simulink model "AFASClosedloopSim"  (R2023a)
settings: Solver=FixedStepAuto  StartTime=0.0  StopTime=600  FixedStep=1/240  RelTol=1e-5
PreLoadFcn:
  | [aircraft, state] = astDehavillandBeaver();
  | thrustX = getCoefficient(aircraft,"CX","Propeller",Component="Propeller");
InitFcn:
  | AFASClosedloopSimInitialization
model workspace (MATLAB code in the model file + MAT data in the model file):
  AirReferencedVelocity = 1
  AircraftPerformance : object (value not decoded)
  CurrentWaypoint = 1
  FCCLatDirMode = 1
  FCCVerticalMode = 1
  FlightPlan = 1
  LookaheadDis = 15
  NextWaypoint = 1
  NumofWaypoint = 1
  OwnshipAircraftID = 1
  PreWaypoint = 1
  PreviousWaypoint : Simulink.Parameter (value not decoded)
  TrajectoryChange = 1
  WaypointType = 1
  inputs0 : object (value not decoded)
  states : object (value not decoded)
  states0 : object (value not decoded)
  other statements: initialize6DOFSkyHogg;
values from neighbouring files (symbols this model uses):
  alt_ft = 1000    [AFASClosedloopSimInitialization.m]
  alt_hold_av = 1.5    [AFASClosedloopSimInitialization.m]
  alt_hold_hold = 0.1    [AFASClosedloopSimInitialization.m]
  alt_hold_vs = 0.58    [AFASClosedloopSimInitialization.m]
  alt_m = 304.8    [AFASClosedloopSimInitialization.m]
  AT_lead_T1 = 1    [AFASClosedloopSimInitialization.m]
  AT_lead_T2 = 1    [AFASClosedloopSimInitialization.m]
  AT_spd_hold_cmpst = 0.5    [AFASClosedloopSimInitialization.m]
  AT_spd_hold_ptch_tau_gain = 0.15    [AFASClosedloopSimInitialization.m]
  AT_spd_hold_rate_damping_gain = 10    [AFASClosedloopSimInitialization.m]
  AT_spd_hold_tas_lp_tau = 5.0    (= 5)    [AFASClosedloopSimInitialization.m]
  AT_spd_hold_tas_val_lp_tau = 0.5    [AFASClosedloopSimInitialization.m]
  AT_struct_den = 1    [AFASClosedloopSimInitialization.m]
  AT_struct_num = 1    [AFASClosedloopSimInitialization.m]
  AT_svo_composite = 1    [AFASClosedloopSimInitialization.m]
  av_hp_fltr_tau = 10    [AFASClosedloopSimInitialization.m]
  av_lp_fltr_tau = 0.5    [AFASClosedloopSimInitialization.m]
  cas_mps = 72.0222    [AFASClosedloopSimInitialization.m]
  Cl0 = 5.910000000000000e-04    (= 0.000591)    [AFASClosedloopSimInitialization.m]
  Cl_beta = -0.0618    [AFASClosedloopSimInitialization.m]
  Cl_da = -0.0992    [AFASClosedloopSimInitialization.m]
  Cl_da_alpha = -0.0827    [AFASClosedloopSimInitialization.m]
  Cl_dr = 0.0069    [AFASClosedloopSimInitialization.m]
  Cl_p = -0.5045    [AFASClosedloopSimInitialization.m]
  Cl_r = 0.1695    [AFASClosedloopSimInitialization.m]
  Cm0 = 0.0945    [AFASClosedloopSimInitialization.m]
  Cm_alpha = -0.6028    [AFASClosedloopSimInitialization.m]
  Cm_alpha2 = -2.1400    (= -2.14)    [AFASClosedloopSimInitialization.m]
  Cm_beta2 = 0.6921    [AFASClosedloopSimInitialization.m]
  Cm_de = -1.9210    (= -1.921)    [AFASClosedloopSimInitialization.m]
  Cm_df = 0.4072    [AFASClosedloopSimInitialization.m]
  Cm_q = -15.5600    (= -15.56)    [AFASClosedloopSimInitialization.m]
  Cm_r = -0.3118    [AFASClosedloopSimInitialization.m]
  Cn0 = -0.0031    [AFASClosedloopSimInitialization.m]
  Cn_beta = 0.0067    [AFASClosedloopSimInitialization.m]
  Cn_beta3 = 0.1373    [AFASClosedloopSimInitialization.m]
  Cn_da = -0.0039    [AFASClosedloopSimInitialization.m]
  Cn_dr = -0.0827    [AFASClosedloopSimInitialization.m]
  Cn_p = -0.1585    [AFASClosedloopSimInitialization.m]
  Cn_q = 0.1595    [AFASClosedloopSimInitialization.m]
  Cn_r = -0.1112    [AFASClosedloopSimInitialization.m]
  Cx0 = -0.0355    [AFASClosedloopSimInitialization.m]
  Cx_alpha = 0.0029    [AFASClosedloopSimInitialization.m]
  Cx_alpha2 = 5.4590    (= 5.459)    [AFASClosedloopSimInitialization.m]
  Cx_alpha3 = -5.1620    (= -5.162)    [AFASClosedloopSimInitialization.m]
  Cx_df = -0.0945    [AFASClosedloopSimInitialization.m]
  Cx_df_alpha = 1.1060    (= 1.106)    [AFASClosedloopSimInitialization.m]
  Cx_dr = 0.0341    [AFASClosedloopSimInitialization.m]
  Cx_q = -0.6748    [AFASClosedloopSimInitialization.m]
  Cy0 = -0.0022    [AFASClosedloopSimInitialization.m]
  Cy_beta = -0.7678    [AFASClosedloopSimInitialization.m]
  Cy_da = -0.0296    [AFASClosedloopSimInitialization.m]
  Cy_dr = 0.1158    [AFASClosedloopSimInitialization.m]
  Cy_dr_alpha = 0.5238    [AFASClosedloopSimInitialization.m]
  Cy_p = -0.1240    (= -0.124)    [AFASClosedloopSimInitialization.m]
  Cy_r = 0.3666    [AFASClosedloopSimInitialization.m]
  Cz0 = -0.0550    (= -0.055)    [AFASClosedloopSimInitialization.m]
  Cz_alpha = -5.5780    (= -5.578)    [AFASClosedloopSimInitialization.m]
  Cz_alpha3 = 3.4420    (= 3.442)    [AFASClosedloopSimInitialization.m]
  Cz_de = -0.3980    (= -0.398)    [AFASClosedloopSimInitialization.m]
  Cz_de_beta = -15.9300    (= -15.93)    [AFASClosedloopSimInitialization.m]
  Cz_df = -1.3770    (= -1.377)    [AFASClosedloopSimInitialization.m]
  Cz_df_alpha = -1.2610    (= -1.261)    [AFASClosedloopSimInitialization.m]
  Cz_q = -2.9880    (= -2.988)    [AFASClosedloopSimInitialization.m]
  hdg_select_hdg_rate_capt = 0.2    [AFASClosedloopSimInitialization.m]
  hdg_select_hdg_rate_damping = 1    [AFASClosedloopSimInitialization.m]
  hdg_select_hdg_rate_track = 0.05    [AFASClosedloopSimInitialization.m]
  lat_accel_aug_lp_tau = 10    [AFASClosedloopSimInitialization.m]
  ltrl_acc_gain = -0.04    [AFASClosedloopSimInitialization.m]
  ltrl_acc_lp_tau = 0.5    [AFASClosedloopSimInitialization.m]
  mach = 0.213    [AFASClosedloopSimInitialization.m]
  OwnshipAircraftConfig = 0    [AFASClosedloopSimInitialization.m]
  pitch_att_gain = 0.7    [AFASClosedloopSimInitialization.m]
  pitch_lead_T1 = 1    [AFASClosedloopSimInitialization.m]
  pitch_lead_T2 = 1    [AFASClosedloopSimInitialization.m]
  pitch_rate_gain = -1400    [AFASClosedloopSimInitialization.m]
  pitch_rate_gain_GAIN1 = -56    [AFASClosedloopSimInitialization.m]
  pitch_rate_gain_GAIN2 = -52.25    [AFASClosedloopSimInitialization.m]
  pitch_rate_gain_IAS1 = 100    [AFASClosedloopSimInitialization.m]
  pitch_rate_gain_IAS2 = 380    [AFASClosedloopSimInitialization.m]
  pitch_rate_gain_schd = [4.24        2.80        2.24        1.68        1.44        1.22        0.97        0.85        0.77        0.72        0.66    ] * 1000    [AFASClosedloopSimInitialization.m]
  pitch_rate_gain_spd = [85          100.0       120.00      140.00      160.00      180.00      200.00      220.00      240.00      260.00      275.00  ] * 0.5144444    [AFASClosedloopSimInitialization.m]
  pitch_schedule_type = 3    [AFASClosedloopSimInitialization.m]
  pitch_struct_den = 1    [AFASClosedloopSimInitialization.m]
  pitch_struct_num = 1    [AFASClosedloopSimInitialization.m]
  pitch_svo_composite = 1    [AFASClosedloopSimInitialization.m]
  pitch_svo_integral = 0.6    [AFASClosedloopSimInitialization.m]
  roll_att_gain = 0.45    [AFASClosedloopSimInitialization.m]
  roll_lead_T1 = 1    [AFASClosedloopSimInitialization.m]
  roll_lead_T2 = 1    [AFASClosedloopSimInitialization.m]
  roll_limit = 30*d2r    (= 0.5235987)    [AFASClosedloopSimInitialization.m]
  roll_rate_gain = 561.5    [AFASClosedloopSimInitialization.m]
  roll_rate_gain_GAIN1 = 57.25    [AFASClosedloopSimInitialization.m]
  roll_rate_gain_GAIN2 = 41.25    [AFASClosedloopSimInitialization.m]
  roll_rate_gain_IAS1 = 100    [AFASClosedloopSimInitialization.m]
  roll_rate_gain_IAS2 = 380    [AFASClosedloopSimInitialization.m]
  roll_rate_gain_schd = [1.30        0.86        0.71        0.63        0.57        0.50        0.46        0.46    ] * 1000    [AFASClosedloopSimInitialization.m]
  roll_rate_gain_spd = [85.00       100.00      120.00      140.00      160.00      200.00      220.00      275.00  ] * 0.5144444    [AFASClosedloopSimInitialization.m]
  roll_schedule_type = 3    [AFASClosedloopSimInitialization.m]
  roll_struct_den = 1    [AFASClosedloopSimInitialization.m]
  roll_struct_num = 1    [AFASClosedloopSimInitialization.m]
  roll_svo_composite = 0.00001    (= 1e-05)    [AFASClosedloopSimInitialization.m]
  roll_svo_integral = 0.6    [AFASClosedloopSimInitialization.m]
  tas_mps = 73.051    [AFASClosedloopSimInitialization.m]
  TGR = 0.25    [AFASClosedloopSimInitialization.m]
  wingrock_enable_alt = 20000    [AFASClosedloopSimInitialization.m]
  wingrock_enable_mach = 0.6    [AFASClosedloopSimInitialization.m]
  wingrock_lookup_data = [2 2  1 1]    [AFASClosedloopSimInitialization.m]
  wingrock_lookup_row = [0 2 5 10]*pi/180    [AFASClosedloopSimInitialization.m]
  wingrock_schedule_type = 3    [AFASClosedloopSimInitialization.m]
  yaw_rate_gain = 15521    [AFASClosedloopSimInitialization.m]
  yaw_rate_gain_GAIN1 = 37.8352    [AFASClosedloopSimInitialization.m]
  yaw_rate_gain_GAIN2 = 24.2654    [AFASClosedloopSimInitialization.m]
  yaw_rate_gain_IAS1 = 100    [AFASClosedloopSimInitialization.m]
  yaw_rate_gain_IAS2 = 340    [AFASClosedloopSimInitialization.m]
  yaw_rate_gain_piecewise_schd = [7.68	5.98		3.22	2.59		1.78 ... (first row only)    [AFASClosedloopSimInitialization.m]
  yaw_rate_gain_schd = [15521    11532   11532   10115   8951.7  7831.7  6829.2  5739.3  4506.7  3317.9  3391.5  2103.9  1404.5  994.3226]    [AFASClosedloopSimInitialization.m]
  yaw_rate_gain_spd = [90       97      106     111     118     127     136     149     165     187     192     228     264     295     ] * 0.5144444    [AFASClosedloopSimInitialization.m]
  yaw_rate_hp_tau = 1.8    [AFASClosedloopSimInitialization.m]
  yd_lead_T1 = yd_a * yd_lead_T2    [AFASClosedloopSimInitialization.m]
  ... (+7 more)
undefined symbols (not defined in the file or in its folder): aircraft, DiscIntNeverNeededParam, Earth, F, Light, MIL, sigbuilder_block, state, WGS84
libraries: aerolibasang x4, aerolibactuator x4, aerolibguid x2, simulink x2, dspnetwork x2, etargetslib x2, shared6dof x1, aerolibadyn x1, aerolibatmos2 x1, aerolibwind2 x1, aerolibtransform2 x1, sharedtransform x1
(part 2 of 4)

== system AFASClosedloopSim/FMGC (Flight Mgt and Guidance & Control)/AFCC: Albatross.ai Flight Control Computer ==
  TMTargets : Inport
  RMTargets : Inport  Port=2
  OwnshipStates : Inport  Port=3
  Bus Selector : BusSelector  OutputSignals=SpdTarget,AltTarget
  Constant : Constant  Value=FCCVerticalMode
  Constant1 : Constant  Value=FCCLatDirMode
  FCC: Mode Logic and Behavior Logic : Subsystem
  FCC: Outerloop & Innerloop Control Laws : Subsystem
  ATServoCmd : Outport
  PitchServoCmd : Outport  Port=2
  RollServoCmd : Outport  Port=3
  YawServoCmd : Outport  Port=4
  wires:
  FCC: Outerloop & Innerloop Control Laws/1(ATServoCmd) -> ATServoCmd/1
  FCC: Outerloop & Innerloop Control Laws/2(PitchServoCmd) -> PitchServoCmd/1
  FCC: Outerloop & Innerloop Control Laws/3(RollSevoCmd) -> RollServoCmd/1
  TMTargets/1 -> Bus Selector/1
  RMTargets/1 -> FCC: Mode Logic and Behavior Logic/3(HDGTarget)
  Bus Selector/1 -> FCC: Mode Logic and Behavior Logic/1(SpdTarget)  "<SpdTarget>"
  Bus Selector/2 -> FCC: Mode Logic and Behavior Logic/2(AltTarget)  "<AltTarget>"
  Constant/1 -> FCC: Mode Logic and Behavior Logic/4(FCCVerticalMode)
  Constant1/1 -> FCC: Mode Logic and Behavior Logic/5(FCCLatDirMode)
  FCC: Mode Logic and Behavior Logic/1(SpdTargetLimited) -> FCC: Outerloop & Innerloop Control Laws/1(SpdTargetLimited)
  FCC: Mode Logic and Behavior Logic/2(AltTargetLimited) -> FCC: Outerloop & Innerloop Control Laws/2(AltTargetLimited)
  FCC: Mode Logic and Behavior Logic/3(HDGTargetLimited) -> FCC: Outerloop & Innerloop Control Laws/3(HDGTargetLimited)
  FCC: Outerloop & Innerloop Control Laws/4(YawServoCmd) -> YawServoCmd/1
  OwnshipStates/1 -> FCC: Outerloop & Innerloop Control Laws/4(OwnshipStates)

== system AFASClosedloopSim/FMGC (Flight Mgt and Guidance & Control)/AFMS: Albatross Flight Management System ==
  OwnshipStates : Inport
  4DTCmd : Inport  Port=2
  Add : Sum  Inputs=+-
  Add1 : Sum  Inputs=+-
  Add2 : Sum  Inputs=+-
  Bus Creator : BusCreator  Inputs=2
  Bus Selector : BusSelector  OutputSignals=Xe,Ye,Ze,u,v,w,psi
  C Caller : CCaller  FunctionName=add  PortSpecificationStruct="%)30     .    6 4   8    (     @         %    \"     ,    !     0         %  0 \"0    $    _    07)G3F%M90  4&]R=$YA;64 4V-O<&4     26YD97@     5'EP90      4VEZ90      27-';&]B86P   X    P    !@    @    $          4    (     0    ,    !         !   P!O=70 #@   #     &    \"     0         !0    @    !     P    $         $  # &]U=  .    .     8    (    !          %    \"     $    &     0         0    !@   $]U='!U=   #@   #@    &    \"     8         !0    @    !     0    $         \"0    @               X    X    !@    @    $          4    (     0    8    !         !     &    9&]U8FQE   .    ,     8    (    !          %    \"     $    !     0         0  $ ,0    X    P    !@    @    ) @        4    (     0    $    !          (  0      #@   #     &    \"     0         !0    @    !     @    $         $  \" '4Q   .    ,     8    (    !          %    \"     $    \"     0         0  ( =3$   X    X    !@    @    $          4    (     0    4    !         !     %    26YP=70    .    .     8    (    !@         %    \"     $    !     0         )    \"               #@   #@    &    \"     0         !0    @    !    !@    $         $     8   !D;W5B;&4   X    P    !@    @    $          4    (     0    $    !         !   0 Q    #@   #     &    \"     D\"        !0    @    !     0    $          @ !       .    ,     8    (    !          %    \"     $    \"     0         0  ( =3(   X    P    !@    @    $          4    (     0    (    !         !   @!U,@  #@   #@    &    \"     0         !0    @    !    !0    $         $     4   !);G!U=     X    X    !@    @    &          4    (     0    $    !          D    (            \\#\\.    .     8    (    !          %    \"     $    &     0         0    !@   &1O=6)L90  #@   #     &    \"     0         !0    @    !     0    $         $  ! #$    .    ,     8    (    \"0(        %    \"     $    !     0         \"  $"
  Calculate Range : aerolibguid/Calculate Range
  Constant : Constant
  Constant1 : Constant
  Current Time : DigitalClock
  CurrentWP : Constant  Value=[117.28257863691368,39.22176648931558,527.0,600]
  Demux : Demux
  Divide : Product  Inputs=*/
  Gain : Gain  Gain=-1
  Mux1 : Mux  Inputs=3
  Mux2 : Mux  Inputs=3
  Scope : Scope
  Scope1 : Scope
  Scope2 : Scope  NumInputPorts=7
  Selector1 : Selector  IndexMode=Zero-based  InputPortWidth=16  IndexOptions=Index vector (port)  Indices=[1]  OutputSizes=1
  Terminator : Terminator
  Trigonometric Function : Trigonometry  Operator=atan2
  WGS84_Location : Subsystem
  TMTargets : Outport
  RMTargets : Outport  Port=2
  wires:
  WGS84_Location/1(x) -> Mux1/1, Add2/1
  OwnshipStates/1 -> Bus Selector/1
  Demux/1 -> WGS84_Location/1(lon)  "<LONGWGS84>"
  Constant/1 -> C Caller/1
  CurrentWP/1 -> Demux/1
  C Caller/1 -> Selector1/2
  Constant1/1 -> C Caller/2
  Demux/2 -> WGS84_Location/2(lat)
  Demux/3 -> Gain/1
  Demux/4 -> Add/1
  Current Time/1 -> Add/2
  Add1/1 -> Trigonometric Function/1
  WGS84_Location/2(y) -> Add1/1, Mux1/2
  Gain/1 -> Bus Creator/2, Mux1/3  "AltTarget"
  Add/1 -> Divide/2, Scope1/1
  Bus Selector/1 -> Add2/2, Mux2/1  "<Xe>"
  Bus Selector/2 -> Mux2/2, Add1/2  "<Ye>"
  Bus Selector/3 -> Mux2/3  "<Ze>"
  Bus Selector/4 -> Scope2/5  "<u>"
  Calculate Range/1 -> Scope2/2, Divide/1
  Bus Selector/5 -> Scope2/4  "<v>"
  Bus Selector/6 -> Scope2/3  "<w>"
  Bus Selector/7 -> Scope2/7  "<psi>"
  Selector1/1 -> Terminator/1
  Mux1/1 -> Calculate Range/1
  Add2/1 -> Trigonometric Function/2
  Mux2/1 -> Calculate Range/2
  Trigonometric Function/1 -> Scope2/1, RMTargets/1
  Divide/1 -> Scope2/6, Bus Creator/1  "SpdTarget"
  Bus Creator/1 -> TMTargets/1

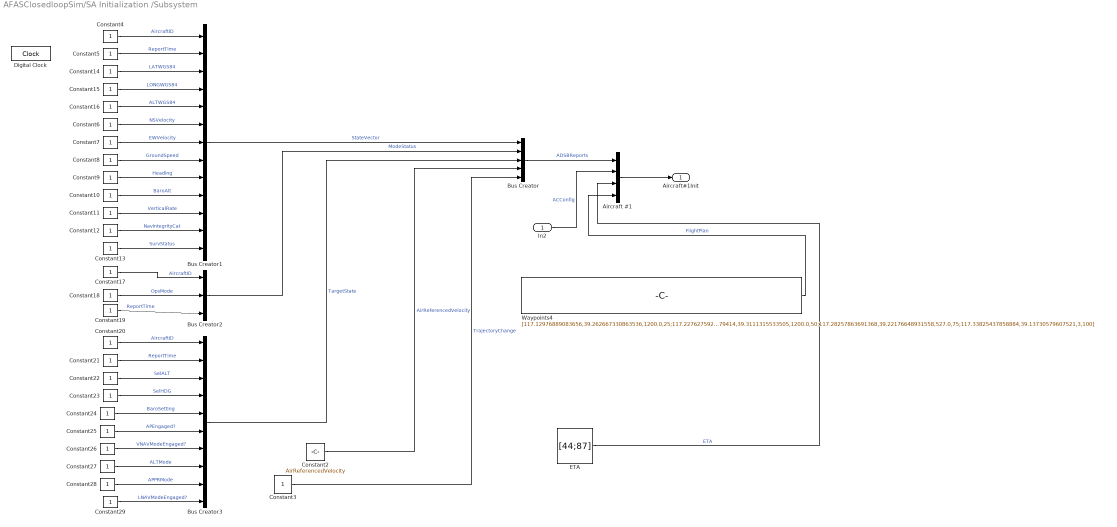
== system AFASClosedloopSim/SA Initialization /Subsystem ==
  In2 : Inport
  Aircraft #1 : BusCreator  Inputs=4
  Bus Creator : BusCreator  Inputs=5
  Bus Creator1 : BusCreator  Inputs=13
  Bus Creator2 : BusCreator  Inputs=3
  Bus Creator3 : BusCreator  Inputs=10
  Constant{3..29} (27 alike) : Constant
  Constant2 : Constant  Value=AirReferencedVelocity
  Digital Clock : DigitalClock
  ETA : Constant  Value=[44;87]
  Waypoints4 : Constant  Value=[117.12976889083656,39.262667330863536,1200.0,25;117.22762759279414,39.3111315533505,1200.0,50;117.28257863691368,39.22176648931558,527.0,75;117.33825437858884,39.13730579607521,3,100]
  Aircraft#1Init : Outport
  wires:
  Constant2/1 -> Bus Creator/4  "AirReferencedVelocity"
  Bus Creator2/1 -> Bus Creator/2  "ModeStatus"
  Bus Creator/1 -> Aircraft #1/1  "ADSBReports"
  In2/1 -> Aircraft #1/2  "ACConfig"
  Bus Creator3/1 -> Bus Creator/3  "TargetState"
  Bus Creator1/1 -> Bus Creator/1  "StateVector"
  Constant3/1 -> Bus Creator/5  "TrajectoryChange"
  Waypoints4/1 -> Aircraft #1/4  "FlightPlan"
  Aircraft #1/1 -> Aircraft#1Init/1
  Constant13/1 -> Bus Creator1/13  "SurvStatus"
  Constant12/1 -> Bus Creator1/12  "NavIntegrityCat"
  Constant11/1 -> Bus Creator1/11  "VerticalRate"
  Constant10/1 -> Bus Creator1/10  "BaroAlt"
  Constant9/1 -> Bus Creator1/9  "Heading"
  Constant8/1 -> Bus Creator1/8  "GroundSpeed"
  Constant7/1 -> Bus Creator1/7  "EWVelocity"
  Constant6/1 -> Bus Creator1/6  "NSVelocity"
  Constant14/1 -> Bus Creator1/3  "LATWGS84"
  Constant5/1 -> Bus Creator1/2  "ReportTime"
  Constant4/1 -> Bus Creator1/1  "AircraftID"
  Constant15/1 -> Bus Creator1/4  "LONGWGS84"
  Constant16/1 -> Bus Creator1/5  "ALTWGS84"
  Constant18/1 -> Bus Creator2/2  "OpsMode"
  Constant17/1 -> Bus Creator2/1  "AircraftID"
  Constant19/1 -> Bus Creator2/3  "ReportTime"
  Constant20/1 -> Bus Creator3/1  "AircraftID"
  Constant21/1 -> Bus Creator3/2  "ReportTime"
  Constant29/1 -> Bus Creator3/10  "LNAVModeEngaged?"
  Constant28/1 -> Bus Creator3/9  "APPRMode"
  Constant27/1 -> Bus Creator3/8  "ALTMode"
  Constant26/1 -> Bus Creator3/7  "VNAVModeEngaged?"
  Constant25/1 -> Bus Creator3/6  "APEngaged?"
  Constant24/1 -> Bus Creator3/5  "BaroSetting"
  Constant23/1 -> Bus Creator3/4  "SelHDG"
  Constant22/1 -> Bus Creator3/3  "SelALT"
  ETA/1 -> Aircraft #1/3  "ETA"

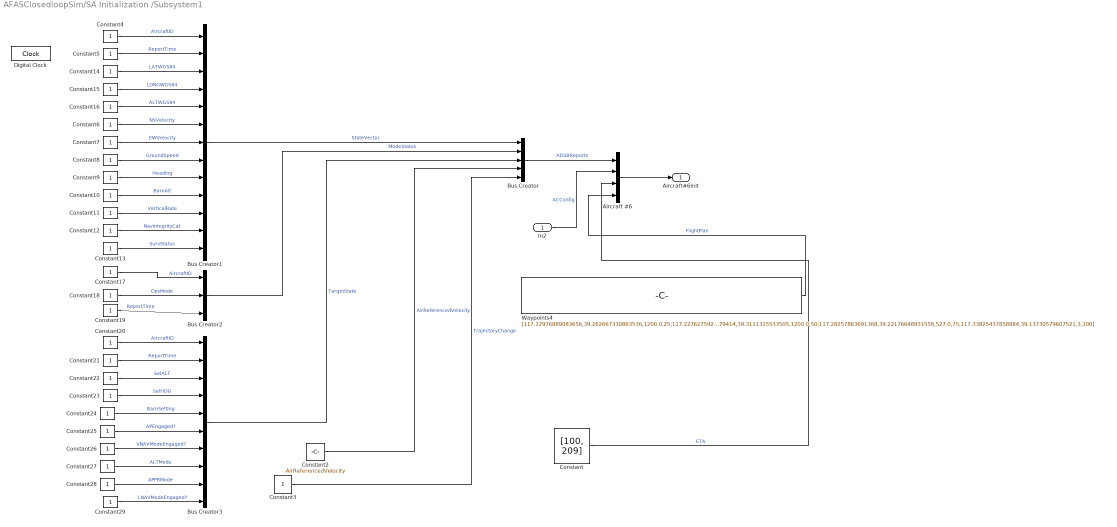
== system AFASClosedloopSim/SA Initialization /Subsystem1 ==
  In2 : Inport
  Aircraft #6 : BusCreator  Inputs=4
  Bus Creator : BusCreator  Inputs=5
  Bus Creator1 : BusCreator  Inputs=13
  Bus Creator2 : BusCreator  Inputs=3
  Bus Creator3 : BusCreator  Inputs=10
  Constant : Constant  Value=[100, 209]
  Constant{3..29} (27 alike) : Constant
  Constant2 : Constant  Value=AirReferencedVelocity
  Digital Clock : DigitalClock
  Waypoints4 : Constant  Value=[117.12976889083656,39.262667330863536,1200.0,25;117.22762759279414,39.3111315533505,1200.0,50;117.28257863691368,39.22176648931558,527.0,75;117.33825437858884,39.13730579607521,3,100]
  Aircraft#6Init : Outport
  wires:
  Constant2/1 -> Bus Creator/4  "AirReferencedVelocity"
  Bus Creator2/1 -> Bus Creator/2  "ModeStatus"
  Bus Creator/1 -> Aircraft #6/1  "ADSBReports"
  In2/1 -> Aircraft #6/2  "ACConfig"
  Bus Creator3/1 -> Bus Creator/3  "TargetState"
  Bus Creator1/1 -> Bus Creator/1  "StateVector"
  Constant3/1 -> Bus Creator/5  "TrajectoryChange"
  Waypoints4/1 -> Aircraft #6/4  "FlightPlan"
  Aircraft #6/1 -> Aircraft#6Init/1
  Constant13/1 -> Bus Creator1/13  "SurvStatus"
  Constant12/1 -> Bus Creator1/12  "NavIntegrityCat"
  Constant11/1 -> Bus Creator1/11  "VerticalRate"
  Constant10/1 -> Bus Creator1/10  "BaroAlt"
  Constant9/1 -> Bus Creator1/9  "Heading"
  Constant8/1 -> Bus Creator1/8  "GroundSpeed"
  Constant7/1 -> Bus Creator1/7  "EWVelocity"
  Constant6/1 -> Bus Creator1/6  "NSVelocity"
  Constant14/1 -> Bus Creator1/3  "LATWGS84"
  Constant5/1 -> Bus Creator1/2  "ReportTime"
  Constant4/1 -> Bus Creator1/1  "AircraftID"
  Constant15/1 -> Bus Creator1/4  "LONGWGS84"
  Constant16/1 -> Bus Creator1/5  "ALTWGS84"
  Constant18/1 -> Bus Creator2/2  "OpsMode"
  Constant17/1 -> Bus Creator2/1  "AircraftID"
  Constant19/1 -> Bus Creator2/3  "ReportTime"
  Constant20/1 -> Bus Creator3/1  "AircraftID"
  Constant21/1 -> Bus Creator3/2  "ReportTime"
  Constant29/1 -> Bus Creator3/10  "LNAVModeEngaged?"
  Constant28/1 -> Bus Creator3/9  "APPRMode"
  Constant27/1 -> Bus Creator3/8  "ALTMode"
  Constant26/1 -> Bus Creator3/7  "VNAVModeEngaged?"
  Constant25/1 -> Bus Creator3/6  "APEngaged?"
  Constant24/1 -> Bus Creator3/5  "BaroSetting"
  Constant23/1 -> Bus Creator3/4  "SelHDG"
  Constant22/1 -> Bus Creator3/3  "SelALT"
  Constant/1 -> Aircraft #6/3  "ETA"

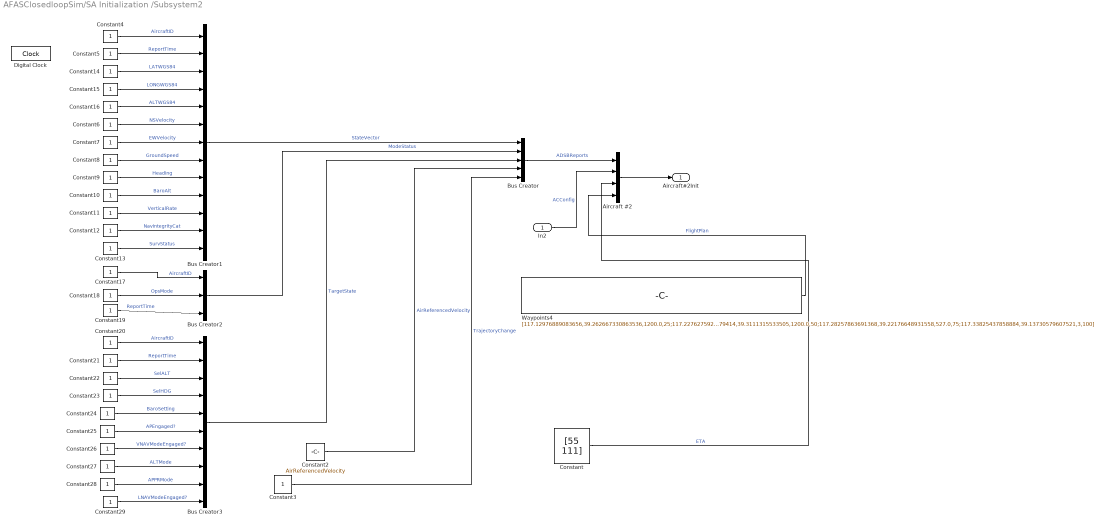
== system AFASClosedloopSim/SA Initialization /Subsystem2 ==
  In2 : Inport
  Aircraft #2 : BusCreator  Inputs=4
  Bus Creator : BusCreator  Inputs=5
  Bus Creator1 : BusCreator  Inputs=13
  Bus Creator2 : BusCreator  Inputs=3
  Bus Creator3 : BusCreator  Inputs=10
  Constant : Constant  Value="[55  111]"
  Constant{3..29} (27 alike) : Constant
  Constant2 : Constant  Value=AirReferencedVelocity
  Digital Clock : DigitalClock
  Waypoints4 : Constant  Value=[117.12976889083656,39.262667330863536,1200.0,25;117.22762759279414,39.3111315533505,1200.0,50;117.28257863691368,39.22176648931558,527.0,75;117.33825437858884,39.13730579607521,3,100]
  Aircraft#2Init : Outport
  wires:
  Constant2/1 -> Bus Creator/4  "AirReferencedVelocity"
  Bus Creator2/1 -> Bus Creator/2  "ModeStatus"
  Bus Creator/1 -> Aircraft #2/1  "ADSBReports"
  In2/1 -> Aircraft #2/2  "ACConfig"
  Bus Creator3/1 -> Bus Creator/3  "TargetState"
  Bus Creator1/1 -> Bus Creator/1  "StateVector"
  Constant3/1 -> Bus Creator/5  "TrajectoryChange"
  Waypoints4/1 -> Aircraft #2/4  "FlightPlan"
  Aircraft #2/1 -> Aircraft#2Init/1
  Constant13/1 -> Bus Creator1/13  "SurvStatus"
  Constant12/1 -> Bus Creator1/12  "NavIntegrityCat"
  Constant11/1 -> Bus Creator1/11  "VerticalRate"
  Constant10/1 -> Bus Creator1/10  "BaroAlt"
  Constant9/1 -> Bus Creator1/9  "Heading"
  Constant8/1 -> Bus Creator1/8  "GroundSpeed"
  Constant7/1 -> Bus Creator1/7  "EWVelocity"
  Constant6/1 -> Bus Creator1/6  "NSVelocity"
  Constant14/1 -> Bus Creator1/3  "LATWGS84"
  Constant5/1 -> Bus Creator1/2  "ReportTime"
  Constant4/1 -> Bus Creator1/1  "AircraftID"
  Constant15/1 -> Bus Creator1/4  "LONGWGS84"
  Constant16/1 -> Bus Creator1/5  "ALTWGS84"
  Constant18/1 -> Bus Creator2/2  "OpsMode"
  Constant17/1 -> Bus Creator2/1  "AircraftID"
  Constant19/1 -> Bus Creator2/3  "ReportTime"
  Constant20/1 -> Bus Creator3/1  "AircraftID"
  Constant21/1 -> Bus Creator3/2  "ReportTime"
  Constant29/1 -> Bus Creator3/10  "LNAVModeEngaged?"
  Constant28/1 -> Bus Creator3/9  "APPRMode"
  Constant27/1 -> Bus Creator3/8  "ALTMode"
  Constant26/1 -> Bus Creator3/7  "VNAVModeEngaged?"
  Constant25/1 -> Bus Creator3/6  "APEngaged?"
  Constant24/1 -> Bus Creator3/5  "BaroSetting"
  Constant23/1 -> Bus Creator3/4  "SelHDG"
  Constant22/1 -> Bus Creator3/3  "SelALT"
  Constant/1 -> Aircraft #2/3  "ETA"

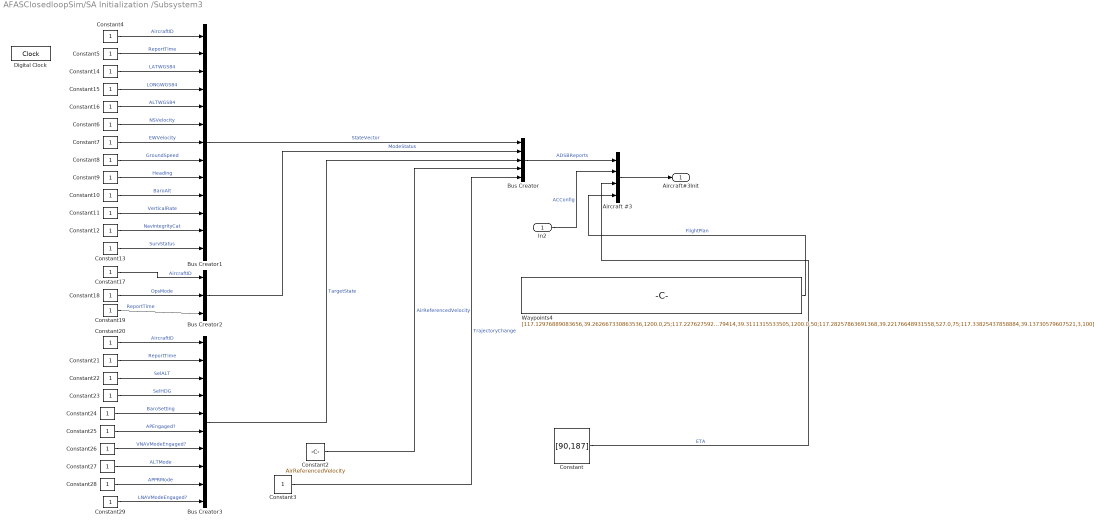
== system AFASClosedloopSim/SA Initialization /Subsystem3 ==
  In2 : Inport
  Aircraft #3 : BusCreator  Inputs=4
  Bus Creator : BusCreator  Inputs=5
  Bus Creator1 : BusCreator  Inputs=13
  Bus Creator2 : BusCreator  Inputs=3
  Bus Creator3 : BusCreator  Inputs=10
  Constant : Constant  Value=[90,187]
  Constant{3..29} (27 alike) : Constant
  Constant2 : Constant  Value=AirReferencedVelocity
  Digital Clock : DigitalClock
  Waypoints4 : Constant  Value=[117.12976889083656,39.262667330863536,1200.0,25;117.22762759279414,39.3111315533505,1200.0,50;117.28257863691368,39.22176648931558,527.0,75;117.33825437858884,39.13730579607521,3,100]
  Aircraft#3Init : Outport
  wires:
  Constant2/1 -> Bus Creator/4  "AirReferencedVelocity"
  Bus Creator2/1 -> Bus Creator/2  "ModeStatus"
  Bus Creator/1 -> Aircraft #3/1  "ADSBReports"
  In2/1 -> Aircraft #3/2  "ACConfig"
  Bus Creator3/1 -> Bus Creator/3  "TargetState"
  Bus Creator1/1 -> Bus Creator/1  "StateVector"
  Constant3/1 -> Bus Creator/5  "TrajectoryChange"
  Waypoints4/1 -> Aircraft #3/4  "FlightPlan"
  Aircraft #3/1 -> Aircraft#3Init/1
  Constant13/1 -> Bus Creator1/13  "SurvStatus"
  Constant12/1 -> Bus Creator1/12  "NavIntegrityCat"
  Constant11/1 -> Bus Creator1/11  "VerticalRate"
  Constant10/1 -> Bus Creator1/10  "BaroAlt"
  Constant9/1 -> Bus Creator1/9  "Heading"
  Constant8/1 -> Bus Creator1/8  "GroundSpeed"
  Constant7/1 -> Bus Creator1/7  "EWVelocity"
  Constant6/1 -> Bus Creator1/6  "NSVelocity"
  Constant14/1 -> Bus Creator1/3  "LATWGS84"
  Constant5/1 -> Bus Creator1/2  "ReportTime"
  Constant4/1 -> Bus Creator1/1  "AircraftID"
  Constant15/1 -> Bus Creator1/4  "LONGWGS84"
  Constant16/1 -> Bus Creator1/5  "ALTWGS84"
  Constant18/1 -> Bus Creator2/2  "OpsMode"
  Constant17/1 -> Bus Creator2/1  "AircraftID"
  Constant19/1 -> Bus Creator2/3  "ReportTime"
  Constant20/1 -> Bus Creator3/1  "AircraftID"
  Constant21/1 -> Bus Creator3/2  "ReportTime"
  Constant29/1 -> Bus Creator3/10  "LNAVModeEngaged?"
  Constant28/1 -> Bus Creator3/9  "APPRMode"
  Constant27/1 -> Bus Creator3/8  "ALTMode"
  Constant26/1 -> Bus Creator3/7  "VNAVModeEngaged?"
  Constant25/1 -> Bus Creator3/6  "APEngaged?"
  Constant24/1 -> Bus Creator3/5  "BaroSetting"
  Constant23/1 -> Bus Creator3/4  "SelHDG"
  Constant22/1 -> Bus Creator3/3  "SelALT"
  Constant/1 -> Aircraft #3/3  "ETA"

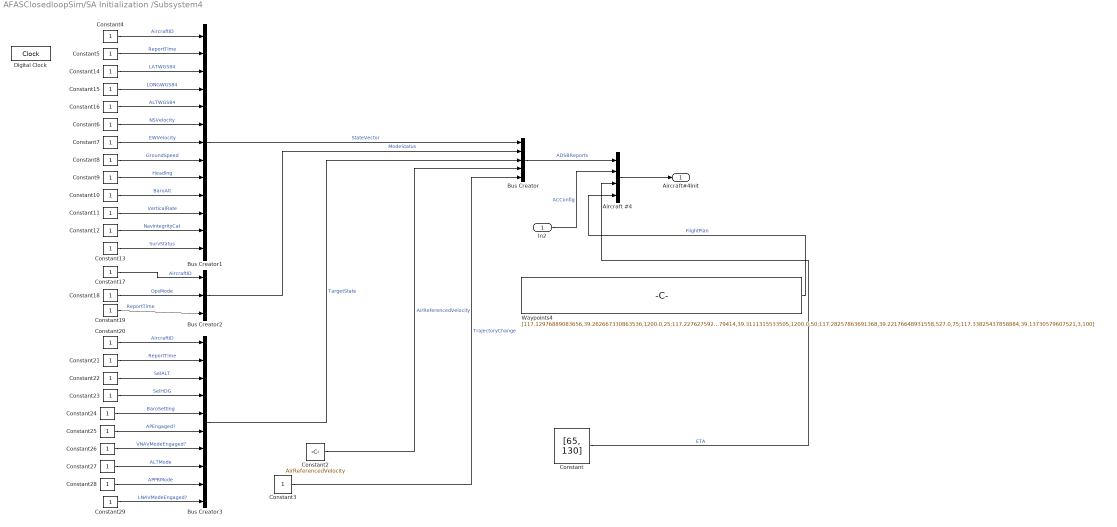
== system AFASClosedloopSim/SA Initialization /Subsystem4 ==
  In2 : Inport
  Aircraft #4 : BusCreator  Inputs=4
  Bus Creator : BusCreator  Inputs=5
  Bus Creator1 : BusCreator  Inputs=13
  Bus Creator2 : BusCreator  Inputs=3
  Bus Creator3 : BusCreator  Inputs=10
  Constant : Constant  Value=[65, 130]
  Constant{3..29} (27 alike) : Constant
  Constant2 : Constant  Value=AirReferencedVelocity
  Digital Clock : DigitalClock
  Waypoints4 : Constant  Value=[117.12976889083656,39.262667330863536,1200.0,25;117.22762759279414,39.3111315533505,1200.0,50;117.28257863691368,39.22176648931558,527.0,75;117.33825437858884,39.13730579607521,3,100]
  Aircraft#4Init : Outport
  wires:
  Constant2/1 -> Bus Creator/4  "AirReferencedVelocity"
  Bus Creator2/1 -> Bus Creator/2  "ModeStatus"
  Bus Creator/1 -> Aircraft #4/1  "ADSBReports"
  In2/1 -> Aircraft #4/2  "ACConfig"
  Bus Creator3/1 -> Bus Creator/3  "TargetState"
  Bus Creator1/1 -> Bus Creator/1  "StateVector"
  Constant3/1 -> Bus Creator/5  "TrajectoryChange"
  Waypoints4/1 -> Aircraft #4/4  "FlightPlan"
  Aircraft #4/1 -> Aircraft#4Init/1
  Constant13/1 -> Bus Creator1/13  "SurvStatus"
  Constant12/1 -> Bus Creator1/12  "NavIntegrityCat"
  Constant11/1 -> Bus Creator1/11  "VerticalRate"
  Constant10/1 -> Bus Creator1/10  "BaroAlt"
  Constant9/1 -> Bus Creator1/9  "Heading"
  Constant8/1 -> Bus Creator1/8  "GroundSpeed"
  Constant7/1 -> Bus Creator1/7  "EWVelocity"
  Constant6/1 -> Bus Creator1/6  "NSVelocity"
  Constant14/1 -> Bus Creator1/3  "LATWGS84"
  Constant5/1 -> Bus Creator1/2  "ReportTime"
  Constant4/1 -> Bus Creator1/1  "AircraftID"
  Constant15/1 -> Bus Creator1/4  "LONGWGS84"
  Constant16/1 -> Bus Creator1/5  "ALTWGS84"
  Constant18/1 -> Bus Creator2/2  "OpsMode"
  Constant17/1 -> Bus Creator2/1  "AircraftID"
  Constant19/1 -> Bus Creator2/3  "ReportTime"
  Constant20/1 -> Bus Creator3/1  "AircraftID"
  Constant21/1 -> Bus Creator3/2  "ReportTime"
  Constant29/1 -> Bus Creator3/10  "LNAVModeEngaged?"
  Constant28/1 -> Bus Creator3/9  "APPRMode"
  Constant27/1 -> Bus Creator3/8  "ALTMode"
  Constant26/1 -> Bus Creator3/7  "VNAVModeEngaged?"
  Constant25/1 -> Bus Creator3/6  "APEngaged?"
  Constant24/1 -> Bus Creator3/5  "BaroSetting"
  Constant23/1 -> Bus Creator3/4  "SelHDG"
  Constant22/1 -> Bus Creator3/3  "SelALT"
  Constant/1 -> Aircraft #4/3  "ETA"

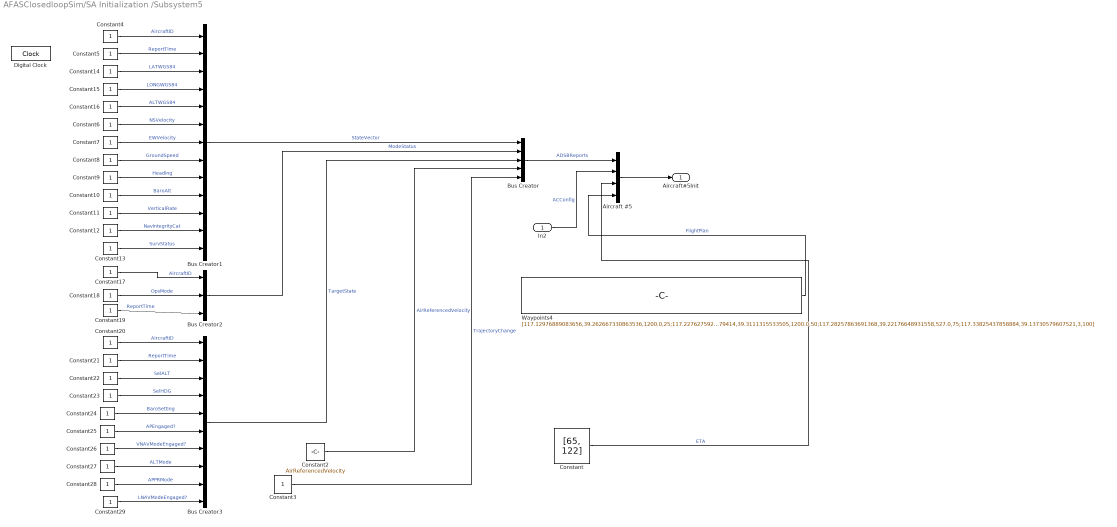
== system AFASClosedloopSim/SA Initialization /Subsystem5 ==
  In2 : Inport
  Aircraft #5 : BusCreator  Inputs=4
  Bus Creator : BusCreator  Inputs=5
  Bus Creator1 : BusCreator  Inputs=13
  Bus Creator2 : BusCreator  Inputs=3
  Bus Creator3 : BusCreator  Inputs=10
  Constant : Constant  Value=[65, 122]
  Constant{3..29} (27 alike) : Constant
  Constant2 : Constant  Value=AirReferencedVelocity
  Digital Clock : DigitalClock
  Waypoints4 : Constant  Value=[117.12976889083656,39.262667330863536,1200.0,25;117.22762759279414,39.3111315533505,1200.0,50;117.28257863691368,39.22176648931558,527.0,75;117.33825437858884,39.13730579607521,3,100]
  Aircraft#5Init : Outport
  wires:
  Constant2/1 -> Bus Creator/4  "AirReferencedVelocity"
  Bus Creator2/1 -> Bus Creator/2  "ModeStatus"
  Bus Creator/1 -> Aircraft #5/1  "ADSBReports"
  In2/1 -> Aircraft #5/2  "ACConfig"
  Bus Creator3/1 -> Bus Creator/3  "TargetState"
  Bus Creator1/1 -> Bus Creator/1  "StateVector"
  Constant3/1 -> Bus Creator/5  "TrajectoryChange"
  Waypoints4/1 -> Aircraft #5/4  "FlightPlan"
  Aircraft #5/1 -> Aircraft#5Init/1
  Constant13/1 -> Bus Creator1/13  "SurvStatus"
  Constant12/1 -> Bus Creator1/12  "NavIntegrityCat"
  Constant11/1 -> Bus Creator1/11  "VerticalRate"
  Constant10/1 -> Bus Creator1/10  "BaroAlt"
  Constant9/1 -> Bus Creator1/9  "Heading"
  Constant8/1 -> Bus Creator1/8  "GroundSpeed"
  Constant7/1 -> Bus Creator1/7  "EWVelocity"
  Constant6/1 -> Bus Creator1/6  "NSVelocity"
  Constant14/1 -> Bus Creator1/3  "LATWGS84"
  Constant5/1 -> Bus Creator1/2  "ReportTime"
  Constant4/1 -> Bus Creator1/1  "AircraftID"
  Constant15/1 -> Bus Creator1/4  "LONGWGS84"
  Constant16/1 -> Bus Creator1/5  "ALTWGS84"
  Constant18/1 -> Bus Creator2/2  "OpsMode"
  Constant17/1 -> Bus Creator2/1  "AircraftID"
  Constant19/1 -> Bus Creator2/3  "ReportTime"
  Constant20/1 -> Bus Creator3/1  "AircraftID"
  Constant21/1 -> Bus Creator3/2  "ReportTime"
  Constant29/1 -> Bus Creator3/10  "LNAVModeEngaged?"
  Constant28/1 -> Bus Creator3/9  "APPRMode"
  Constant27/1 -> Bus Creator3/8  "ALTMode"
  Constant26/1 -> Bus Creator3/7  "VNAVModeEngaged?"
  Constant25/1 -> Bus Creator3/6  "APEngaged?"
  Constant24/1 -> Bus Creator3/5  "BaroSetting"
  Constant23/1 -> Bus Creator3/4  "SelHDG"
  Constant22/1 -> Bus Creator3/3  "SelALT"
  Constant/1 -> Aircraft #5/3  "ETA"

== system AFASClosedloopSim/Servo/Aileron: Actuation System Model ==
  ailMotorPosCmd_rad : Inport
  Aileron: Nonlinear Second-Order Actuator : aerolibactuator/Nonlinear Second-Order Actuator  wn_fin=1  z_fin=0.3  fin_max=20*pi/180  fin_min=-20*pi/180  fin_maxrate=500*pi/180  fin_act_0=0  fin_act_vel=0
  Gear Ratio Drum to Ail : Gain  Gain=0.2428
  Gear Ratio Motor to Drum : Gain  Gain=1/TGR
  Scope1 : Scope
  Scope2 : Scope
  Scope3 : Scope
  tAilPos_rad : Outport
  wires:
  Gear Ratio Drum to Ail/1 -> Scope3/1, tAilPos_rad/1
  Gear Ratio Motor to Drum/1 -> Gear Ratio Drum to Ail/1
  ailMotorPosCmd_rad/1 -> Scope2/1, Aileron: Nonlinear Second-Order Actuator/1
  Aileron: Nonlinear Second-Order Actuator/1 -> Scope1/1, Gear Ratio Motor to Drum/1

== system AFASClosedloopSim/Servo/Elevator: Actuation System Model ==
  motorPosCmd_rad : Inport
  Elevator: Nonlinear Second-Order Actuator : aerolibactuator/Nonlinear Second-Order Actuator  wn_fin=1  z_fin=0.3  fin_max=20*pi/180  fin_min=-20*pi/180  fin_maxrate=500*pi/180  fin_act_0=0  fin_act_vel=0
  Gear Ratio Drum to Elev : Gain  Gain=0.1439
  Gear Ratio Motor to Drum : Gain  Gain=1/TGR
  elevPos_rad : Outport
  wires:
  Elevator: Nonlinear Second-Order Actuator/1 -> Gear Ratio Motor to Drum/1
  Gear Ratio Motor to Drum/1 -> Gear Ratio Drum to Elev/1
  motorPosCmd_rad/1 -> Elevator: Nonlinear Second-Order Actuator/1
  Gear Ratio Drum to Elev/1 -> elevPos_rad/1

== system AFASClosedloopSim/Servo/Rudder: Actuation System Model ==
  rudMotorPosCmd_rad : Inport
  Gear Ratio Drum to Rud : Gain  Gain=0.3977
  Gear Ratio Motor to Drum1 : Gain  Gain=1/TGR
  Rudder: Nonlinear Second-Order Actuator : aerolibactuator/Nonlinear Second-Order Actuator  wn_fin=1  z_fin=0.3  fin_max=20*pi/180  fin_min=-20*pi/180  fin_maxrate=500*pi/180  fin_act_0=0  fin_act_vel=0
  rudPos_rad : Outport
  wires:
  rudMotorPosCmd_rad/1 -> Rudder: Nonlinear Second-Order Actuator/1
  Gear Ratio Motor to Drum1/1 -> Gear Ratio Drum to Rud/1
  Rudder: Nonlinear Second-Order Actuator/1 -> Gear Ratio Motor to Drum1/1
  Gear Ratio Drum to Rud/1 -> rudPos_rad/1

== system AFASClosedloopSim/6 DoF Airframe Model/Aerodynamic Model/Actuator Increments ==
  alpha : Inport  Unit=rad
  beta : Inport  Port=2  Unit=rad
  ActuatorCmds : Inport  Port=3  Unit=rad
  Aileron : Subsystem
  Elevator : Subsystem
  Flap : Subsystem
  Flap Deflections : Constant  Value=0
  Mux : Mux  Inputs=2
  Rudder : Subsystem
  Sum : Sum  Inputs=++++  InputSameDT=on  SaturateOnIntegerOverflow=on  OutDataTypeStr=Inherit: Same as first input
  Coefficients : Outport  VectorParamsAs1DForOutWhenUnconnected=off
  wires:
  alpha/1 -> Flap/1(Alpha), Rudder/1(Alpha), Aileron/1(alpha)
  beta/1 -> Elevator/2(Beta)
  Aileron/1(delCoeff) -> Sum/1
  Elevator/1(delCoeff) -> Sum/2
  Rudder/1(delCoeff) -> Sum/3
  Flap/1(delCoeff) -> Sum/4
  Sum/1 -> Coefficients/1
  ActuatorCmds/1 -> Mux/1
  Flap Deflections/1 -> Mux/2  "FlapCmd"
  Mux/1 -> Aileron/2(Actuators), Elevator/1(Actuators), Rudder/2(Actuators), Flap/2(Actuators)

== system AFASClosedloopSim/6 DoF Airframe Model/Aerodynamic Model/Body Rate Damping ==
  V : Inport  Unit=m/second
  p,q,r : Inport  Port=2  Unit=rad/second
  Bus Selector : BusSelector  OutputSignals=p_wind,q_wind,r_wind
  Product : Product  InputSameDT=on  SaturateOnIntegerOverflow=on  OutDataTypeStr=Inherit: Same as first input
  Product1 : Product  InputSameDT=on  SaturateOnIntegerOverflow=on  OutDataTypeStr=Inherit: Same as first input
  Product2 : Product  InputSameDT=on  SaturateOnIntegerOverflow=on  OutDataTypeStr=Inherit: Same as first input
  Product3 : Product  Inputs=*/  InputSameDT=on  SaturateOnIntegerOverflow=on  OutDataTypeStr=Inherit: Same as first input
  Reference Length : Gain  Gain=aircraft.ReferenceLength  SaturateOnIntegerOverflow=on  OutDataTypeStr=Inherit: Same as input  ParamDataTypeStr=Inherit: Same as input
  Reference Span : Gain  Gain=aircraft.ReferenceSpan/2  SaturateOnIntegerOverflow=on  OutDataTypeStr=Inherit: Same as input  ParamDataTypeStr=Inherit: Same as input
  "Reference Span " : Gain  Gain=aircraft.ReferenceSpan/2  SaturateOnIntegerOverflow=on  OutDataTypeStr=Inherit: Same as input  ParamDataTypeStr=Inherit: Same as input
  Sum1 : Sum  Inputs=+++  InputSameDT=on  SaturateOnIntegerOverflow=on  OutDataTypeStr=Inherit: Same as first input
  p : Subsystem
  q : Subsystem
  r : Subsystem
  Coefficients : Outport  VectorParamsAs1DForOutWhenUnconnected=off
  wires:
  p/1(delCoeff) -> Product/1
  q/1(delCoeff) -> Product1/1
  p,q,r/1 -> Bus Selector/1
  Sum1/1 -> Product3/1
  V/1 -> Product3/2
  Product3/1 -> Coefficients/1
  Product1/1 -> Reference Length/1
  Product2/1 -> "Reference Span "/1
  Product/1 -> Reference Span/1
  r/1(delCoeff) -> Product2/1
  Reference Length/1 -> Sum1/2
  Reference Span/1 -> Sum1/1
  "Reference Span "/1 -> Sum1/3
  Bus Selector/1 -> Product/2  "<p_wind>"
  Bus Selector/2 -> Product1/2  "<q_wind>"
  Bus Selector/3 -> Product2/2  "<r_wind>"

== system AFASClosedloopSim/6 DoF Airframe Model/Aerodynamic Model/Datum Coefficients ==
  alpha : Inport  Unit=radian
  beta : Inport  Port=2  Unit=radian
  Constant : Constant  Value=[Cx0,Cy0,Cz0,Cl0,Cm0,Cn0]
  Gain : Gain  Gain=Cx_alpha  SaturateOnIntegerOverflow=on  OutDataTypeStr=Inherit: Same as input  ParamDataTypeStr=Inherit: Same as input
  Gain1 : Gain  Gain=Cx_alpha2  SaturateOnIntegerOverflow=on  OutDataTypeStr=Inherit: Same as input  ParamDataTypeStr=Inherit: Same as input
  Gain10 : Gain  Gain=Cm_alpha2  SaturateOnIntegerOverflow=on  OutDataTypeStr=Inherit: Same as input  ParamDataTypeStr=Inherit: Same as input
  Gain11 : Gain  Gain=Cm_beta2  SaturateOnIntegerOverflow=on  OutDataTypeStr=Inherit: Same as input  ParamDataTypeStr=Inherit: Same as input
  Gain2 : Gain  Gain=Cx_alpha3  SaturateOnIntegerOverflow=on  OutDataTypeStr=Inherit: Same as input  ParamDataTypeStr=Inherit: Same as input
  Gain3 : Gain  Gain=Cy_beta  SaturateOnIntegerOverflow=on  OutDataTypeStr=Inherit: Same as input  ParamDataTypeStr=Inherit: Same as input
  Gain4 : Gain  Gain=Cz_alpha  SaturateOnIntegerOverflow=on  OutDataTypeStr=Inherit: Same as input  ParamDataTypeStr=Inherit: Same as input
  Gain5 : Gain  Gain=Cz_alpha3  SaturateOnIntegerOverflow=on  OutDataTypeStr=Inherit: Same as input  ParamDataTypeStr=Inherit: Same as input
  Gain6 : Gain  Gain=Cl_beta  SaturateOnIntegerOverflow=on  OutDataTypeStr=Inherit: Same as input  ParamDataTypeStr=Inherit: Same as input
  Gain7 : Gain  Gain=Cn_beta  SaturateOnIntegerOverflow=on  OutDataTypeStr=Inherit: Same as input  ParamDataTypeStr=Inherit: Same as input
  Gain8 : Gain  Gain=Cn_beta3  SaturateOnIntegerOverflow=on  OutDataTypeStr=Inherit: Same as input  ParamDataTypeStr=Inherit: Same as input
  Gain9 : Gain  Gain=Cm_alpha  SaturateOnIntegerOverflow=on  OutDataTypeStr=Inherit: Same as input  ParamDataTypeStr=Inherit: Same as input
  Mux1 : Mux  Inputs=6
  Product{1..4} (4 alike) : Product  InputSameDT=on  SaturateOnIntegerOverflow=on  OutDataTypeStr=Inherit: Same as first input
  Sum : Sum  Inputs=+++  SaturateOnIntegerOverflow=on
  Sum1 : Sum  SaturateOnIntegerOverflow=on
  Sum2 : Sum  SaturateOnIntegerOverflow=on
  Sum3 : Sum  Inputs=+++  SaturateOnIntegerOverflow=on
  Sum4 : Sum  Inputs=|++  SaturateOnIntegerOverflow=on
  Coefficients : Outport  VectorParamsAs1DForOutWhenUnconnected=off
  wires:
  Constant/1 -> Sum4/2
  Sum4/1 -> Coefficients/1
  Mux1/1 -> Sum4/1
  Gain10/1 -> Sum3/2
  Product2/1 -> Product3/1, Gain11/1
  Gain11/1 -> Sum3/3
  Gain9/1 -> Sum3/1
  Sum3/1 -> Mux1/5  "Cm"
  Product3/1 -> Gain8/1
  Gain8/1 -> Sum2/2
  Gain7/1 -> Sum2/1
  Gain5/1 -> Sum1/1
  Gain4/1 -> Sum1/2
  Product1/1 -> Gain5/1, Gain2/1
  Gain2/1 -> Sum/3
  Product4/1 -> Product1/1, Gain10/1, Gain1/1
  Gain1/1 -> Sum/2
  Gain/1 -> Sum/1
  Sum2/1 -> Mux1/6  "Cn"
  Sum/1 -> Mux1/1  "Cx"
  Sum1/1 -> Mux1/3  "Cz"
  Gain3/1 -> Mux1/2  "Cy"
  Gain6/1 -> Mux1/4  "Cl"
  alpha/1 -> Product1/2, Product4/2, Product4/1, Gain/1, Gain9/1, Gain4/1
  beta/1 -> Gain6/1, Gain3/1, Product3/2, Gain7/1, Product2/2, Product2/1

== system AFASClosedloopSim/6 DoF Airframe Model/Aerodynamic Model/Subsystem ==
  Vb : Inport
  "Incidence, Sideslip, & Airspeed" : aerolibasang/Incidence, Sideslip, & Airspeed
  Product{,1..3} (4 alike) : Product
  Alpha : Outport
  Alpha2 : Outport  Port=2
  Alpha3 : Outport  Port=3
  Beta : Outport  Port=4
  Beta2 : Outport  Port=5
  Beta3 : Outport  Port=6
  V : Outport  Port=7
  wires:
  Product/1 -> Product1/1, Alpha2/1
  "Incidence, Sideslip, & Airspeed"/1 -> Product/1, Alpha/1, Product/2, Product1/2
  "Incidence, Sideslip, & Airspeed"/3 -> V/1
  Vb/1 -> "Incidence, Sideslip, & Airspeed"/1
  Product1/1 -> Alpha3/1
  Product2/1 -> Product3/1, Beta2/1
  Product3/1 -> Beta3/1
  "Incidence, Sideslip, & Airspeed"/2 -> Product3/2, Product2/2, Product2/1, Beta/1

== system AFASClosedloopSim/6 DoF Airframe Model/Aerodynamic Model/ToBus ==
  I : Inport
  Bus Creator3 : BusCreator  Inputs=3
  Demux : Demux  Outputs=3
  O : Outport  VectorParamsAs1DForOutWhenUnconnected=off
  wires:
  I/1 -> Demux/1
  Demux/2 -> Bus Creator3/2  "q_wind"
  Bus Creator3/1 -> O/1
  Demux/3 -> Bus Creator3/3  "r_wind"
  Demux/1 -> Bus Creator3/1  "p_wind"

== system AFASClosedloopSim/AFAS has four sub-moduels: 1) Detect and Avoid (DAA); 2) Aircraft Separation Assurance System (ASAS); 3) Collaborative Decision Assistance System (CDAS); 4) Decentralized Decision Assistance System (DDAS) /DDAS: Decentralized Decision Assistance System/If Action Subsystem1 ==
  FlightRules : Inport
  OwnshipStates : Inport  Port=2
  SituationAwarness : Inport  Port=3
  OwnshipInformation : Inport  Port=4
  Action Port : ActionPort  ActionPortLabel=if(u1 ~= 1)
  Bus Selector : BusSelector  OutputSignals=Aircraft#1Init.ETA,Aircraft#2Init.ETA,Aircraft#3Init.ETA,Aircraft#4Init.ETA,Aircraft#5Init.ETA,Aircraft#6Init.ETA
  Bus Selector1 : BusSelector  OutputSignals=ETA
  Constant : Constant  Value=[10,20]
  Delay : Delay  DelayLength=1
  Display : Display
  Matrix Concatenate : Concatenate  NumInputs=6  Mode=Multidimensional array  ConcatenateDimension=2
  Optimize Function : MATLAB Function  TreatAsAtomicUnit=on
  ETASchedulingDecision : Outport
  OptimizedSequence : Outport  Port=2
  wires:
  SituationAwarness/1 -> Bus Selector/1
  Bus Selector/1 -> Matrix Concatenate/1  "<ETA>"
  Bus Selector/2 -> Matrix Concatenate/2  "<ETA>"
  Bus Selector/3 -> Matrix Concatenate/3  "<ETA>"
  Optimize Function/1(t) -> ETASchedulingDecision/1
  OwnshipInformation/1 -> Bus Selector1/1
  Bus Selector/6 -> Matrix Concatenate/6  "<ETA>"
  Bus Selector/5 -> Matrix Concatenate/5  "<ETA>"
  Bus Selector/4 -> Matrix Concatenate/4  "<ETA>"
  Constant/1 -> Optimize Function/1(separationTime)
  Matrix Concatenate/1 -> Display/1, Optimize Function/3(AwarenessETA)
  Bus Selector1/1 -> Optimize Function/4(ownshipETA)  "<ETA>"
  Optimize Function/2(s) -> OptimizedSequence/1
  Optimize Function/3(over) -> Delay/1
  Delay/1 -> Optimize Function/2(data)

== system AFASClosedloopSim/AFAS has four sub-moduels: 1) Detect and Avoid (DAA); 2) Aircraft Separation Assurance System (ASAS); 3) Collaborative Decision Assistance System (CDAS); 4) Decentralized Decision Assistance System (DDAS) /DDAS: Decentralized Decision Assistance System/Ownship Aircraft 4DT Command ==
  ETASchedulingDecision : Inport
  SituationAwarness : Inport  Port=2
  OwnshipInformation : Inport  Port=3
  AircraftConfiguration : Constant  Value=[1;1;1;1;1;1]
  Bus Selector : BusSelector  OutputSignals=Aircraft#1Init.FlightPlan,Aircraft#2Init.FlightPlan,Aircraft#3Init.FlightPlan,Aircraft#4Init.FlightPlan,Aircraft#5Init.FlightPlan,Aircraft#6Init.FlightPlan
  Bus Selector1 : BusSelector  OutputSignals=ETA,FlightPlan
  C Caller : CCaller  FunctionName=incrementElement  PortSpecificationStruct="%)30     .    @ 4   8    (     @         %    \"     ,    !     0         %  0 \"0    $    _    07)G3F%M90  4&]R=$YA;64 4V-O<&4     26YD97@     5'EP90      4VEZ90      27-';&]B86P   X    P    !@    @    $          4    (     0    $    !         !   0!U    #@   #     &    \"     0         !0    @    !     0    $         $  ! '4    .    0     8    (    !          %    \"     $    +     0         0    \"P   $EN<'5T3W5T<'5T       .    .     8    (    !@         %    \"     $    !     0         )    \"               #@   #@    &    \"     0         !0    @    !    !0    $         $     4   !I;G0S,@    X    P    !@    @    $          4    (     0    (    !         !   @ M,0  #@   #     &    \"     D\"        !0    @    !     0    $          @ !       .    ,     8    (    !          %    \"     $    $     0         0  0 <VEZ90X    P    !@    @    $          4    (     0    0    !         !  ! !S:7IE#@   #@    &    \"     0         !0    @    !    !0    $         $     4   !);G!U=     X    X    !@    @    &          4    (     0    $    !          D    (            \\#\\.    .     8    (    !          %    \"     $    &     0         0    !@   '5I;G0S,@  #@   #     &    \"     0         !0    @    !     0    $         $  ! #$    .    ,     8    (    \"0(        %    \"     $    !     0         \"  $       X   !     !@    @    $          4    (     0    T    !         !     -    :6YC<F5M96YT7VED>     X   !     !@    @    $          4    (     0    T    !         !     -    :6YC<F5M96YT7VED>     X    X    !@    @    $          4    (     0    4    !         !     %    26YP=70    .    .     8    (    !@         %    \"     $    !     0         )    \"             ! #@   #@    &    \"     0         !0    @    !    !@    $         $     8   !U:6YT,S(   X    P    !@    @    $          4    (     0    $    !         !   0 Q    #@   #     &    \"     D\"        !0    @    !     0    $          @ !"
  AIAircraft4DTCmd : Outport
  ownship4DTCmd : Outport  Port=2
  wires:
  ETASchedulingDecision/1 -> ?
  ? -> ownship4DTCmd/1
  ? -> AIAircraft4DTCmd/1
  SituationAwarness/1 -> Bus Selector/1
  OwnshipInformation/1 -> Bus Selector1/1

== system AFASClosedloopSim/AFAS has four sub-moduels: 1) Detect and Avoid (DAA); 2) Aircraft Separation Assurance System (ASAS); 3) Collaborative Decision Assistance System (CDAS); 4) Decentralized Decision Assistance System (DDAS) /DDAS: Decentralized Decision Assistance System/WGS84_Location ==
  lon : Inport
  lat : Inport  Port=2
  alt : Inport  Port=3
  C Caller : CCaller  FunctionName=latToMeters  PortSpecificationStruct="%)30     .    6 4   8    (     @         %    \"     ,    !     0         %  0 \"0    $    _    07)G3F%M90  4&]R=$YA;64 4V-O<&4     26YD97@     5'EP90      4VEZ90      27-';&]B86P   X    P    !@    @    $          4    (     0    ,    !         !   P!O=70 #@   #     &    \"     0         !0    @    !     P    $         $  # &]U=  .    .     8    (    !          %    \"     $    &     0         0    !@   $]U='!U=   #@   #@    &    \"     8         !0    @    !     0    $         \"0    @               X    X    !@    @    $          4    (     0    8    !         !     &    9&]U8FQE   .    ,     8    (    !          %    \"     $    !     0         0  $ ,0    X    P    !@    @    ) @        4    (     0    $    !          (  0      #@   #     &    \"     0         !0    @    !    !     $         $  $ &QA=#$.    ,     8    (    !          %    \"     $    $     0         0  0 ;&%T,0X    X    !@    @    $          4    (     0    4    !         !     %    26YP=70    .    .     8    (    !@         %    \"     $    !     0         )    \"               #@   #@    &    \"     0         !0    @    !    !@    $         $     8   !D;W5B;&4   X    P    !@    @    $          4    (     0    $    !         !   0 Q    #@   #     &    \"     D\"        !0    @    !     0    $          @ !       .    ,     8    (    !          %    \"     $    $     0         0  0 ;&%T,@X    P    !@    @    $          4    (     0    0    !         !  ! !L870R#@   #@    &    \"     0         !0    @    !    !0    $         $     4   !);G!U=     X    X    !@    @    &          4    (     0    $    !          D    (            \\#\\.    .     8    (    !          %    \"     $    &     0         0    !@   &1O=6)L90  #@   #     &    \"     0         !0    @    !     0    $         $  ! #$    .    ,     8    (    \"0(        %    \"     $    !     0         \"  $"
  C Caller1 : CCaller  FunctionName=lonToMeters  PortSpecificationStruct="%)30     .    ^ 8   8    (     @         %    \"     0    !     0         %  0 \"0    $    _    07)G3F%M90  4&]R=$YA;64 4V-O<&4     26YD97@     5'EP90      4VEZ90      27-';&]B86P   X    P    !@    @    $          4    (     0    ,    !         !   P!O=70 #@   #     &    \"     0         !0    @    !     P    $         $  # &]U=  .    .     8    (    !          %    \"     $    &     0         0   ...(+2020 chars)"
  lat1 : Constant  Value=39.1682
  lon1 : Constant  Value=116.8277
  x : Outport
  y : Outport  Port=2
  z : Outport  Port=3
  wires:
  lon1/1 -> C Caller1/2
  lon/1 -> C Caller1/1
  alt/1 -> z/1
  lat1/1 -> C Caller/2, C Caller1/3
  lat/1 -> C Caller/1
  C Caller/1 -> y/1
  C Caller1/1 -> x/1

== system AFASClosedloopSim/FMGC (Flight Mgt and Guidance & Control)/AFCC: Albatross.ai Flight Control Computer/FCC: Mode Logic and Behavior Logic ==
  SpdTarget : Inport
  AltTarget : Inport  Port=2
  HDGTarget : Inport  Port=3
  FCCVerticalMode : Inport  Port=4
  FCCLatDirMode : Inport  Port=5
  Terminator : Terminator
  Terminator1 : Terminator
  SpdTargetLimited : Outport
  AltTargetLimited : Outport  Port=2
  HDGTargetLimited : Outport  Port=3
  wires:
  FCCVerticalMode/1 -> Terminator/1
  FCCLatDirMode/1 -> Terminator1/1
  SpdTarget/1 -> SpdTargetLimited/1
  AltTarget/1 -> AltTargetLimited/1
  HDGTarget/1 -> HDGTargetLimited/1
